simulink model "myproject_exec"  (Simulink 3.00)
undefined symbols (not defined in the file): RPi, W1_owscfg
libraries: execlib x9

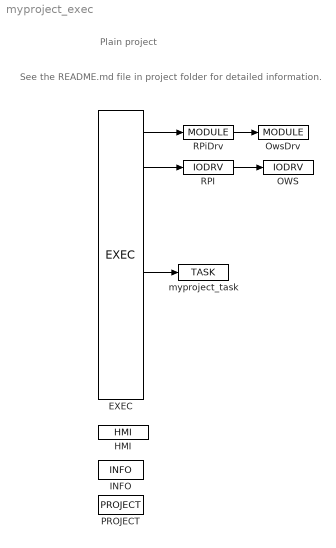
== system myproject_exec ==
  note: Plain project
  note: See the README.md file in project
      | folder for detailed information.
  EXEC : execlib/EXEC  target=Generic target device  tick=0.05  ntick0=2  ntick1=50  ntick2=100  ntick3=1200  pri0=5  pri1=9  pri2=13  pri3=18
  HMI : execlib/HMI  IncludeHMI=off  HmiDir=hmi  SourceDir=hmisrc  GenerateWebWatch=off  GenerateRexHMI=off  RedirectToHMI=off  Compression=on
  INFO : execlib/INFO  Title=OwsDrv_Aliases  Author=Gizmo  Description=How to change One Wire Sensor/Actuator path from outside of OwsDrv.  Customer=Rexygen Studio Example
  OWS : execlib/IODRV  module=OwsDrv  classname=OwsDrv  cfgname=RPi-W1_owscfg.rio  factor=6  stack=10240  pri=3  timer=off
  OwsDrv : execlib/MODULE
  PROJECT : execlib/PROJECT  SourcesOnTarget=off
  RPI : execlib/IODRV  module=RPiDrv  classname=RPiDrv  factor=1  stack=10240  pri=3  timer=off
  RPiDrv : execlib/MODULE
  myproject_task : execlib/TASK  factor=1  start=0  stop=1  stack=10240  MDLOPEN=on
  wires:
  EXEC/1 -> RPiDrv/1
  EXEC/2 -> RPI/1
  EXEC/5 -> myproject_task/1
  RPI/1 -> OWS/1
  RPiDrv/1 -> OwsDrv/1
